simulink model "afe_rst_inv_psm_distributed_control_two_delays"  (R2025b)
settings: Solver=ode1be  StartTime=0.0  StopTime=simlength  FixedStep=tc  MaxStep=Tc
undefined symbols (not defined in the file): Adrso, Amplitude_U, Amplitude_V, Amplitude_W, Aresd, b, Bresd, CFi, CFu, Cresd, Crso, CTRPIFF_CLIP_RELEASE, dead_time_INV, emf_fb_p, emf_fb_p_ccaller_1, emf_fb_p_ccaller_2, emf_p, emf_p_ccaller_1, emf_p_ccaller_2, end_time_LVRT, fPWM_INV, g0_161Hz, g0_500Hz, g1_161Hz, g1_500Hz, i_grid_neg_eta_lim, i_grid_neg_eta_red_lim, i_grid_neg_xi_lim, i_grid_neg_xi_red_lim, i_grid_pos_eta_lim, i_grid_pos_eta_red_lim, ibez, id_lim, ieta_neg_ref_lim, ieta_pos_ref_lim, Igrid_phase_normalization_factor, iq_lim, ixi_pos_ref_lim, Jm, Jm_norm, k_frt_ref, kg, ki_afe, ki_i, ki_id, ki_iq, ki_rc_neg_grid, ki_rc_pos_grid, ki_vs, ki_w, kp_afe, kp_i, kp_id, kp_iq, kp_rc_neg_grid, kp_rc_pos_grid, kp_vs, kp_w, kw, l1 ... (+47)
libraries: fl_lib x145, nesl_utility x81, simulink x11, cstblocks x7, single_phase_transformer_lib x3, flexshaft_lib x1, pmsm_uvw_with_harmonics_lib x1
(part 8 of 15)

== system afe_rst_inv_psm_distributed_control_two_delays/mainboard_afe/voltage_sequence_avg/Moving Average Filter2/Reset Trigger ==
  Clock : Clock
  Constant1 : Constant  Value=simlength
  Constant3 : Constant  Value=0
  Constant4 : Constant
  Mod : Math  Operator=mod
  Switch : Switch  Criteria=u2 ~= 0  SaturateOnIntegerOverflow=off  InputSameDT=off
  Zero-Order Hold : ZeroOrderHold  SampleTime=ts_afe
  Out1 : Outport
  wires:
  Constant3/1 -> Switch/1
  Zero-Order Hold/1 -> Mod/1
  Constant4/1 -> Switch/3
  Mod/1 -> Switch/2
  Clock/1 -> Zero-Order Hold/1
  Switch/1 -> Out1/1  "Reset"
  Constant1/1 -> Mod/2

== system afe_rst_inv_psm_distributed_control_two_delays/mainboard_afe/voltage_sequence_avg/Moving Average Filter3/Enabled Subsystem ==
  In1 : Inport
  Enable : EnablePort
  Constant2 : Constant
  Divide : Product  Inputs=*/
  Gain1 : Gain  Gain=1/(2*pi)
  Gain9 : Gain  Gain=2
  Zero-Order Hold : ZeroOrderHold  SampleTime=ts_afe
  Out1 : Outport
  wires:
  Gain1/1 -> Gain9/1
  Zero-Order Hold/1 -> Out1/1  "period"
  Gain9/1 -> Divide/2
  In1/1 -> Gain1/1  "Omega_el"
  Divide/1 -> Zero-Order Hold/1
  Constant2/1 -> Divide/1

== system afe_rst_inv_psm_distributed_control_two_delays/mainboard_afe/voltage_sequence_avg/Moving Average Filter3/Reset Trigger ==
  Clock : Clock
  Constant1 : Constant  Value=simlength
  Constant3 : Constant  Value=0
  Constant4 : Constant
  Mod : Math  Operator=mod
  Switch : Switch  Criteria=u2 ~= 0  SaturateOnIntegerOverflow=off  InputSameDT=off
  Zero-Order Hold : ZeroOrderHold  SampleTime=ts_afe
  Out1 : Outport
  wires:
  Constant1/1 -> Mod/2
  Switch/1 -> Out1/1  "Reset"
  Clock/1 -> Zero-Order Hold/1
  Mod/1 -> Switch/2
  Constant4/1 -> Switch/3
  Zero-Order Hold/1 -> Mod/1
  Constant3/1 -> Switch/1

== system afe_rst_inv_psm_distributed_control_two_delays/mainboard_afe/voltage_sequence_avg/Moving Average Filter4/Enabled Subsystem ==
  In1 : Inport
  Enable : EnablePort
  Constant2 : Constant
  Divide : Product  Inputs=*/
  Gain1 : Gain  Gain=1/(2*pi)
  Gain9 : Gain  Gain=2
  Zero-Order Hold : ZeroOrderHold  SampleTime=ts_afe
  Out1 : Outport
  wires:
  Constant2/1 -> Divide/1
  Divide/1 -> Zero-Order Hold/1
  In1/1 -> Gain1/1  "Omega_el"
  Gain9/1 -> Divide/2
  Zero-Order Hold/1 -> Out1/1  "period"
  Gain1/1 -> Gain9/1

== system afe_rst_inv_psm_distributed_control_two_delays/mainboard_afe/voltage_sequence_avg/Moving Average Filter4/Reset Trigger ==
  Clock : Clock
  Constant1 : Constant  Value=simlength
  Constant3 : Constant  Value=0
  Constant4 : Constant
  Mod : Math  Operator=mod
  Switch : Switch  Criteria=u2 ~= 0  SaturateOnIntegerOverflow=off  InputSameDT=off
  Zero-Order Hold : ZeroOrderHold  SampleTime=ts_afe
  Out1 : Outport
  wires:
  Constant3/1 -> Switch/1
  Zero-Order Hold/1 -> Mod/1
  Constant4/1 -> Switch/3
  Mod/1 -> Switch/2
  Clock/1 -> Zero-Order Hold/1
  Switch/1 -> Out1/1  "Reset"
  Constant1/1 -> Mod/2

== system afe_rst_inv_psm_distributed_control_two_delays/AFE-Modular/afe_leg_a/driver_board_a/current_ctrl/phase_current_control ==
  In1 : Inport
  is_abc : Inport  Port=2
  Bus Creator1 : BusCreator  Inputs=2
  Bus Creator2 : BusCreator  Inputs=3
  Bus Selector1 : BusSelector  OutputSignals=usa_ctrl,usb_ctrl,usc_ctrl
  MATLAB Function : MATLAB Function  TreatAsAtomicUnit=on
  Selector : Selector  InputPortWidth=3  IndexOptions=Index vector (dialog)  Indices=1  OutputSizes=1
  Unit Delay2 : UnitDelay  SampleTime=ts_afe  HasFrameUpgradeWarning=on
  Unit Delay3 : UnitDelay  SampleTime=ts_afe  HasFrameUpgradeWarning=on
  isa_ref/isa : Scope  NumInputPorts=2
      settings: SampleTime=ts_afe  ActiveDisplayYMinimum=-1.14664  ActiveDisplayYMaximum=1.21003
  phase-current-control-dba : Subsystem
  us_alphabeta_ctrl : Outport  VectorParamsAs1DForOutWhenUnconnected=off
  tag scope: usa_ctrl_dba=global
  wires:
  Bus Creator1/1 -> us_alphabeta_ctrl/1
  Unit Delay2/1 -> Bus Creator1/1  "us_alpha_ctrl"
  Bus Selector1/1 -> MATLAB Function/1(a)  "<usa_ctrl>"
  MATLAB Function/2(beta) -> Unit Delay3/1
  Bus Selector1/2 -> MATLAB Function/2(b)  "<usb_ctrl>"
  Unit Delay3/1 -> Bus Creator1/2  "us_beta_ctrl"
  MATLAB Function/1(alpha) -> Unit Delay2/1
  Bus Selector1/3 -> MATLAB Function/3(c)  "<usc_ctrl>"
  phase-current-control-dba/1(Out1) -> [usa_ctrl_dba], Bus Creator2/1  "usa_ctrl"
  is_abc/1 -> phase-current-control-dba/2(is_abc), isa_ref/isa/2  "isa"
  In1/1 -> Selector/1
  [usb_ctrl_dbb_fb_dba] -> Bus Creator2/2  "usb_ctrl"
  [usc_ctrl_dbc_fb_dba] -> Bus Creator2/3  "usc_ctrl"
  Bus Creator2/1 -> Bus Selector1/1  "us_abc_ctrl"
  Selector/1 -> phase-current-control-dba/1(In1), isa_ref/isa/1  "isa_ref"

== system afe_rst_inv_psm_distributed_control_two_delays/AFE-Modular/afe_leg_a/driver_board_a/current_ctrl/xieta2abc ==
  pos_xi : Inport
  pos_eta : Inport  Port=2
  neg_xi : Inport  Port=3
  neg_eta : Inport  Port=4
  gamma : Inport  Port=5
  MATLAB Function2 : MATLAB Function  TreatAsAtomicUnit=on
  Mux : Mux  Inputs=3
  Negative Sequence : MATLAB Function  TreatAsAtomicUnit=on
  Positive Sequence : MATLAB Function  TreatAsAtomicUnit=on
  Sum : Sum  Inputs=|++
  Sum1 : Sum  Inputs=|++
  i_abc : Outport
  wires:
  Mux/1 -> i_abc/1  "i_abc"
  pos_eta/1 -> Positive Sequence/2(eta)
  pos_xi/1 -> Positive Sequence/1(xi)
  neg_xi/1 -> Negative Sequence/1(xi)
  Sum1/1 -> MATLAB Function2/2(beta)
  MATLAB Function2/2(b) -> Mux/2  "i_b"
  Negative Sequence/2(beta) -> Sum1/2
  Positive Sequence/1(alpha) -> Sum/1
  Negative Sequence/1(alpha) -> Sum/2
  MATLAB Function2/3(c) -> Mux/3  "i_c"
  gamma/1 -> Positive Sequence/3(gamma), Negative Sequence/3(gamma)
  Sum/1 -> MATLAB Function2/1(alpha)
  Positive Sequence/2(beta) -> Sum1/1
  MATLAB Function2/1(a) -> Mux/1  "i_a"
  neg_eta/1 -> Negative Sequence/2(eta)

== system afe_rst_inv_psm_distributed_control_two_delays/AFE-Modular/afe_leg_a/driver_board_a/dq_pll/pll_stageA ==
  gamma_grid : Inport
  Math Function : Math  Operator=magnitude^2  SignedPower=on
  Math Function1 : Math  Operator=magnitude^2  SignedPower=on
  Reciprocal Sqrt : Sqrt  Operator=rSqrt
  Saturation : Saturate  UpperLimit=inf  LowerLimit=0.02
  Sum : Sum  Inputs=|++
  sequences : Subsystem
  transformation : Subsystem
  u_grid_pos_xi : Outport  VectorParamsAs1DForOutWhenUnconnected=off
  u_grid_pos_eta : Outport  Port=2  VectorParamsAs1DForOutWhenUnconnected=off
  tag scope: ugrid_unorm_phase_a=global
  wires:
  transformation/1(ug_alpha) -> Math Function/1, sequences/1(u_grid_alpha)
  transformation/2(ug_beta) -> Math Function1/1, sequences/2(u_grid_beta)
  Math Function/1 -> Sum/1
  Math Function1/1 -> Sum/2
  Sum/1 -> Saturation/1
  Reciprocal Sqrt/1 -> [ugrid_unorm_phase_a]
  Saturation/1 -> Reciprocal Sqrt/1
  gamma_grid/1 -> sequences/3(gamma_grid)
  sequences/1(u_grid_pos_xi) -> u_grid_pos_xi/1
  sequences/2(u_grid_pos_eta) -> u_grid_pos_eta/1
  [ugb_pu_dbb_fb_dba] -> transformation/2(ug_b)
  [uga_pu_dba] -> transformation/1(ug_a)
  [ugc_pu_dbc_fb_dba] -> transformation/3(ug_c)

== system afe_rst_inv_psm_distributed_control_two_delays/AFE-Modular/afe_leg_a/driver_board_a/dq_pll/pll_stageB ==
  u_grid_pos_xi : Inport
  u_grid_pos_eta : Inport  Port=2
  -2<x<2 : Saturate  UpperLimit=2  LowerLimit=-2
  Constant4 : Constant  Value=omega_grid_nom
  Product1 : Product  RndMeth=Zero
  Product2 : Product  RndMeth=Zero
  Sum3 : Sum  SaturateOnIntegerOverflow=on
  Sum4 : Sum  SaturateOnIntegerOverflow=on
  Sum5 : Sum  Inputs=++|
  Unit Delay{1..5} (5 alike) : UnitDelay  SampleTime=ts_afe  HasFrameUpgradeWarning=on
  bounder1 : MATLAB Function  TreatAsAtomicUnit=on  SystemSampleTime=ts_afe
  kp : Gain  Gain=pll_i1*ts_afe  SaturateOnIntegerOverflow=on  OutDataTypeStr=Inherit: Same as input  ParamDataTypeStr=Inherit: Same as input
  kp1 : Gain  Gain=pll_p  SaturateOnIntegerOverflow=on  OutDataTypeStr=Inherit: Same as input  ParamDataTypeStr=Inherit: Same as input
  kp2 : Gain  Gain=ts_afe  SaturateOnIntegerOverflow=on  OutDataTypeStr=Inherit: Same as input  ParamDataTypeStr=Inherit: Same as input
  gamma_grid_pll : Outport  VectorParamsAs1DForOutWhenUnconnected=off
  wires:
  Unit Delay4/1 -> Sum5/2, Sum3/2
  Sum3/1 -> -2<x<2/1
  Sum4/1 -> bounder1/1(u)
  Unit Delay1/1 -> Sum4/2
  -2<x<2/1 -> Unit Delay4/1  "i1"
  kp2/1 -> Sum4/1
  Constant4/1 -> Product2/2
  [ugrid_unorm_phase_a] -> Unit Delay3/1
  kp/1 -> Sum3/1
  Sum5/1 -> Product2/1
  bounder1/1(y) -> Unit Delay1/1, Unit Delay2/1
  u_grid_pos_eta/1 -> Unit Delay5/1
  Product2/1 -> kp2/1
  Product1/1 -> kp/1, kp1/1  "V l"
  kp1/1 -> Sum5/1
  Unit Delay2/1 -> gamma_grid_pll/1
  Unit Delay3/1 -> Product1/2
  Unit Delay5/1 -> Product1/1

== system afe_rst_inv_psm_distributed_control_two_delays/AFE-Modular/afe_leg_a/driver_board_a/voltage-current-acquisition/is_eta_neg_ref_fieldbus ==
  is : Inport
  Unit Delay : UnitDelay  SampleTime=ts_afe  HasFrameUpgradeWarning=on
  Unit Delay1 : UnitDelay  SampleTime=ts_afe  HasFrameUpgradeWarning=on
  Zero-Order Hold : ZeroOrderHold  SampleTime=ts_afe
  is_fb : Outport
  wires:
  is/1 -> Zero-Order Hold/1
  Unit Delay/1 -> Unit Delay1/1
  Zero-Order Hold/1 -> Unit Delay/1
  Unit Delay1/1 -> is_fb/1

== system afe_rst_inv_psm_distributed_control_two_delays/AFE-Modular/afe_leg_a/driver_board_a/voltage-current-acquisition/is_eta_pos_ref_fieldbus ==
  is : Inport
  Unit Delay : UnitDelay  SampleTime=ts_afe  HasFrameUpgradeWarning=on
  Unit Delay1 : UnitDelay  SampleTime=ts_afe  HasFrameUpgradeWarning=on
  Zero-Order Hold : ZeroOrderHold  SampleTime=ts_afe
  is_fb : Outport
  wires:
  is/1 -> Zero-Order Hold/1
  Unit Delay/1 -> Unit Delay1/1
  Zero-Order Hold/1 -> Unit Delay/1
  Unit Delay1/1 -> is_fb/1

== system afe_rst_inv_psm_distributed_control_two_delays/AFE-Modular/afe_leg_a/driver_board_a/voltage-current-acquisition/is_xi_neg_ref_fieldbus ==
  is : Inport
  Unit Delay : UnitDelay  SampleTime=ts_afe  HasFrameUpgradeWarning=on
  Unit Delay1 : UnitDelay  SampleTime=ts_afe  HasFrameUpgradeWarning=on
  Zero-Order Hold : ZeroOrderHold  SampleTime=ts_afe
  is_fb : Outport
  wires:
  Unit Delay/1 -> Unit Delay1/1
  Zero-Order Hold/1 -> Unit Delay/1
  is/1 -> Zero-Order Hold/1
  Unit Delay1/1 -> is_fb/1

== system afe_rst_inv_psm_distributed_control_two_delays/AFE-Modular/afe_leg_a/driver_board_a/voltage-current-acquisition/isa_measure ==
  is : Inport
  Gain : Gain  Gain=1/Igrid_phase_normalization_factor
  Quantizer : Quantizer  QuantizationInterval=CurrentQuantization
  Unit Delay : UnitDelay  SampleTime=ts_afe  HasFrameUpgradeWarning=on
  Zero-Order Hold : ZeroOrderHold  SampleTime=ts_afe
  is_pu : Outport
  wires:
  Quantizer/1 -> Zero-Order Hold/1
  Gain/1 -> is_pu/1
  Zero-Order Hold/1 -> Unit Delay/1
  Unit Delay/1 -> Gain/1
  is/1 -> Quantizer/1

== system afe_rst_inv_psm_distributed_control_two_delays/AFE-Modular/afe_leg_a/driver_board_a/voltage-current-acquisition/isb_fieldbus ==
  is : Inport
  Unit Delay : UnitDelay  SampleTime=ts_afe  HasFrameUpgradeWarning=on
  Unit Delay1 : UnitDelay  SampleTime=ts_afe  HasFrameUpgradeWarning=on
  Zero-Order Hold : ZeroOrderHold  SampleTime=ts_afe
  is_fb : Outport
  wires:
  is/1 -> Zero-Order Hold/1
  Unit Delay/1 -> Unit Delay1/1
  Zero-Order Hold/1 -> Unit Delay/1
  Unit Delay1/1 -> is_fb/1

== system afe_rst_inv_psm_distributed_control_two_delays/AFE-Modular/afe_leg_a/driver_board_a/voltage-current-acquisition/isc_fieldbus ==
  is : Inport
  Unit Delay : UnitDelay  SampleTime=ts_afe  HasFrameUpgradeWarning=on
  Unit Delay1 : UnitDelay  SampleTime=ts_afe  HasFrameUpgradeWarning=on
  Zero-Order Hold : ZeroOrderHold  SampleTime=ts_afe
  is_fb : Outport
  wires:
  is/1 -> Zero-Order Hold/1
  Unit Delay/1 -> Unit Delay1/1
  Zero-Order Hold/1 -> Unit Delay/1
  Unit Delay1/1 -> is_fb/1

== system afe_rst_inv_psm_distributed_control_two_delays/AFE-Modular/afe_leg_a/driver_board_a/voltage-current-acquisition/ixi_ref_fieldbus ==
  is : Inport
  Unit Delay : UnitDelay  SampleTime=ts_afe  HasFrameUpgradeWarning=on
  Unit Delay1 : UnitDelay  SampleTime=ts_afe  HasFrameUpgradeWarning=on
  Zero-Order Hold : ZeroOrderHold  SampleTime=ts_afe
  is_fb : Outport
  wires:
  is/1 -> Zero-Order Hold/1
  Unit Delay/1 -> Unit Delay1/1
  Zero-Order Hold/1 -> Unit Delay/1
  Unit Delay1/1 -> is_fb/1

== system afe_rst_inv_psm_distributed_control_two_delays/AFE-Modular/afe_leg_a/driver_board_a/voltage-current-acquisition/ixi_ref_fieldbus1 ==
  is : Inport
  Unit Delay : UnitDelay  SampleTime=ts_afe  HasFrameUpgradeWarning=on
  Unit Delay1 : UnitDelay  SampleTime=ts_afe  HasFrameUpgradeWarning=on
  Zero-Order Hold : ZeroOrderHold  SampleTime=ts_afe
  is_fb : Outport
  wires:
  is/1 -> Zero-Order Hold/1
  Unit Delay/1 -> Unit Delay1/1
  Zero-Order Hold/1 -> Unit Delay/1
  Unit Delay1/1 -> is_fb/1

== system afe_rst_inv_psm_distributed_control_two_delays/AFE-Modular/afe_leg_a/driver_board_a/voltage-current-acquisition/ub_ctrl_fieldbus ==
  u_ctrl : Inport
  Unit Delay : UnitDelay  SampleTime=ts_afe  HasFrameUpgradeWarning=on
  Unit Delay1 : UnitDelay  SampleTime=ts_afe  HasFrameUpgradeWarning=on
  Zero-Order Hold : ZeroOrderHold  SampleTime=ts_afe
  u_ctrl_fb : Outport
  wires:
  u_ctrl/1 -> Zero-Order Hold/1
  Unit Delay/1 -> Unit Delay1/1
  Zero-Order Hold/1 -> Unit Delay/1
  Unit Delay1/1 -> u_ctrl_fb/1

== system afe_rst_inv_psm_distributed_control_two_delays/AFE-Modular/afe_leg_a/driver_board_a/voltage-current-acquisition/uc_ctrl_fieldbus ==
  u_ctrl : Inport
  Unit Delay : UnitDelay  SampleTime=ts_afe  HasFrameUpgradeWarning=on
  Unit Delay1 : UnitDelay  SampleTime=ts_afe  HasFrameUpgradeWarning=on
  Zero-Order Hold : ZeroOrderHold  SampleTime=ts_afe
  u_ctrl_fb : Outport
  wires:
  Zero-Order Hold/1 -> Unit Delay/1
  u_ctrl/1 -> Zero-Order Hold/1
  Unit Delay/1 -> Unit Delay1/1
  Unit Delay1/1 -> u_ctrl_fb/1

== system afe_rst_inv_psm_distributed_control_two_delays/AFE-Modular/afe_leg_a/driver_board_a/voltage-current-acquisition/uga_measure ==
  ug : Inport
  Gain : Gain  Gain=1/V_phase_normalization_factor
  Quantizer : Quantizer  QuantizationInterval=CurrentQuantization
  Unit Delay : UnitDelay  SampleTime=ts_afe  HasFrameUpgradeWarning=on
  Zero-Order Hold : ZeroOrderHold  SampleTime=ts_afe
  ug_pu : Outport
  wires:
  ug/1 -> Quantizer/1
  Unit Delay/1 -> Gain/1
  Zero-Order Hold/1 -> Unit Delay/1
  Gain/1 -> ug_pu/1
  Quantizer/1 -> Zero-Order Hold/1

== system afe_rst_inv_psm_distributed_control_two_delays/AFE-Modular/afe_leg_a/driver_board_a/voltage-current-acquisition/ugb_fieldbus ==
  ug : Inport
  Unit Delay : UnitDelay  SampleTime=ts_afe  HasFrameUpgradeWarning=on
  Unit Delay1 : UnitDelay  SampleTime=ts_afe  HasFrameUpgradeWarning=on
  Zero-Order Hold : ZeroOrderHold  SampleTime=ts_afe
  ug_fb : Outport
  wires:
  ug/1 -> Zero-Order Hold/1
  Zero-Order Hold/1 -> Unit Delay/1
  Unit Delay/1 -> Unit Delay1/1
  Unit Delay1/1 -> ug_fb/1

== system afe_rst_inv_psm_distributed_control_two_delays/AFE-Modular/afe_leg_a/driver_board_a/voltage-current-acquisition/ugc_fieldbus ==
  ug : Inport
  Unit Delay : UnitDelay  SampleTime=ts_afe  HasFrameUpgradeWarning=on
  Unit Delay1 : UnitDelay  SampleTime=ts_afe  HasFrameUpgradeWarning=on
  Zero-Order Hold : ZeroOrderHold  SampleTime=ts_afe
  ug_fb : Outport
  wires:
  ug/1 -> Zero-Order Hold/1
  Unit Delay/1 -> Unit Delay1/1
  Zero-Order Hold/1 -> Unit Delay/1
  Unit Delay1/1 -> ug_fb/1

== system afe_rst_inv_psm_distributed_control_two_delays/AFE-Modular/afe_leg_a/modulator/sv_pwm/modulator ==
  u : Inport
  v : Inport  Port=2
  w : Inport  Port=3
  Bus Creator : BusCreator  Inputs=6
  PWM generator 1 : Subsystem  mask{f=fPWM_INV, ph=0, m_up=0.98, m_low=0.02, dead_time=dead_time_INV, vg_firing=15, polarity=1}
      mask prompts: f "Frequency"; ph "Phase"; m_up "Max Input Modulation Value"; m_low "Min Input Modulation Value"; dead_time "Dead Time"; vg_firing "Gate Voltage"
  PWM generator 2 : Subsystem  mask{f=fPWM_INV, ph=0, m_up=0.98, m_low=0.02, dead_time=dead_time_INV, vg_firing=15, polarity=1}
      mask prompts: f "Frequency"; ph "Phase"; m_up "Max Input Modulation Value"; m_low "Min Input Modulation Value"; dead_time "Dead Time"; vg_firing "Gate Voltage"
  PWM generator 3 : Subsystem  mask{f=fPWM_INV, ph=0, m_up=0.98, m_low=0.02, dead_time=dead_time_INV, vg_firing=15, polarity=1}
      mask prompts: f "Frequency"; ph "Phase"; m_up "Max Input Modulation Value"; m_low "Min Input Modulation Value"; dead_time "Dead Time"; vg_firing "Gate Voltage"
  firing_gates : Outport
  wires:
  u/1 -> PWM generator 1/1(m_index)
  w/1 -> PWM generator 3/1(m_index)
  v/1 -> PWM generator 2/1(m_index)
  PWM generator 1/2(m2) -> Bus Creator/2  "pwm_u_bottom"
  Bus Creator/1 -> firing_gates/1
  PWM generator 2/1(m1) -> Bus Creator/3  "pwm_v_top"
  PWM generator 3/1(m1) -> Bus Creator/5  "pwm_w_top"
  PWM generator 2/2(m2) -> Bus Creator/4  "pwm_v_bottom"
  PWM generator 3/2(m2) -> Bus Creator/6  "pwm_w_bottom"
  PWM generator 1/1(m1) -> Bus Creator/1  "pwm_u_top"

== system afe_rst_inv_psm_distributed_control_two_delays/AFE-Modular/afe_leg_b/driver_board_b/current_ctrl/phase_current_control ==
  In1 : Inport
  is_abc : Inport  Port=2
  Bus Creator1 : BusCreator  Inputs=2
  Bus Creator2 : BusCreator  Inputs=3
  Bus Selector1 : BusSelector  OutputSignals=usa_ctrl,usb_ctrl,usc_ctrl
  MATLAB Function : MATLAB Function  TreatAsAtomicUnit=on
  Selector : Selector  InputPortWidth=3  IndexOptions=Index vector (dialog)  Indices=2  OutputSizes=1
  Unit Delay2 : UnitDelay  SampleTime=ts_afe  HasFrameUpgradeWarning=on
  Unit Delay3 : UnitDelay  SampleTime=ts_afe  HasFrameUpgradeWarning=on
  isb_ref/isb : Scope  NumInputPorts=2
      settings: SampleTime=ts_afe  ActiveDisplayYMinimum=-2.19741  ActiveDisplayYMaximum=6.15124
  phase-current-control-dbb : Subsystem
  us_alphabeta_ctrl : Outport  VectorParamsAs1DForOutWhenUnconnected=off
  tag scope: usb_ctrl_dbb=global
  wires:
  Bus Creator1/1 -> us_alphabeta_ctrl/1
  Unit Delay2/1 -> Bus Creator1/1  "us_alpha_ctrl"
  Bus Selector1/1 -> MATLAB Function/1(a)  "<usa_ctrl>"
  MATLAB Function/2(beta) -> Unit Delay3/1
  Bus Selector1/2 -> MATLAB Function/2(b)  "<usb_ctrl>"
  Unit Delay3/1 -> Bus Creator1/2  "us_beta_ctrl"
  MATLAB Function/1(alpha) -> Unit Delay2/1
  Bus Selector1/3 -> MATLAB Function/3(c)  "<usc_ctrl>"
  is_abc/1 -> phase-current-control-dbb/2(is_abc), isb_ref/isb/2  "isb"
  In1/1 -> Selector/1
  [usc_ctrl_dbc_fb_dbb] -> Bus Creator2/3  "usc_ctrl"
  phase-current-control-dbb/1(Out1) -> [usb_ctrl_dbb], Bus Creator2/2  "usb_ctrl"
  [usa_ctrl_dba_fb_dbb] -> Bus Creator2/1  "usa_ctrl"
  Bus Creator2/1 -> Bus Selector1/1  "us_abc_ctrl"
  Selector/1 -> phase-current-control-dbb/1(In1), isb_ref/isb/1  "isb_ref"

== system afe_rst_inv_psm_distributed_control_two_delays/AFE-Modular/afe_leg_b/driver_board_b/current_ctrl/xieta2abc ==
  pos_xi : Inport
  pos_eta : Inport  Port=2
  neg_xi : Inport  Port=3
  neg_eta : Inport  Port=4
  gamma : Inport  Port=5
  MATLAB Function2 : MATLAB Function  TreatAsAtomicUnit=on
  Mux : Mux  Inputs=3
  Negative Sequence : MATLAB Function  TreatAsAtomicUnit=on
  Positive Sequence : MATLAB Function  TreatAsAtomicUnit=on
  Sum : Sum  Inputs=|++
  Sum1 : Sum  Inputs=|++
  i_abc_reference : Outport
  wires:
  Mux/1 -> i_abc_reference/1  "i_abc_reference"
  pos_eta/1 -> Positive Sequence/2(eta)
  pos_xi/1 -> Positive Sequence/1(xi)
  neg_xi/1 -> Negative Sequence/1(xi)
  Sum1/1 -> MATLAB Function2/2(beta)
  MATLAB Function2/2(b) -> Mux/2  "i_b"
  Negative Sequence/2(beta) -> Sum1/2
  Positive Sequence/1(alpha) -> Sum/1
  Negative Sequence/1(alpha) -> Sum/2
  MATLAB Function2/3(c) -> Mux/3  "i_c"
  gamma/1 -> Positive Sequence/3(gamma), Negative Sequence/3(gamma)
  Sum/1 -> MATLAB Function2/1(alpha)
  Positive Sequence/2(beta) -> Sum1/1
  MATLAB Function2/1(a) -> Mux/1  "i_a"
  neg_eta/1 -> Negative Sequence/2(eta)

== system afe_rst_inv_psm_distributed_control_two_delays/AFE-Modular/afe_leg_b/driver_board_b/dq_pll/pll_stageA ==
  gamma_grid : Inport
  Math Function : Math  Operator=magnitude^2  SignedPower=on
  Math Function1 : Math  Operator=magnitude^2  SignedPower=on
  Reciprocal Sqrt : Sqrt  Operator=rSqrt
  Saturation : Saturate  UpperLimit=inf  LowerLimit=0.02
  Sum : Sum  Inputs=|++
  mormalization_and_transformation : Subsystem
  sequences : Subsystem
  u_grid_pos_xi : Outport  VectorParamsAs1DForOutWhenUnconnected=off
  u_grid_pos_eta : Outport  Port=2  VectorParamsAs1DForOutWhenUnconnected=off
  tag scope: ugrid_unorm_phase_b=global
  wires:
  mormalization_and_transformation/1(ug_alpha) -> Math Function/1, sequences/1(u_grid_alpha)
  mormalization_and_transformation/2(ug_beta) -> Math Function1/1, sequences/2(u_grid_beta)
  Math Function/1 -> Sum/1
  Math Function1/1 -> Sum/2
  Sum/1 -> Saturation/1
  Reciprocal Sqrt/1 -> [ugrid_unorm_phase_b]
  Saturation/1 -> Reciprocal Sqrt/1
  gamma_grid/1 -> sequences/3(gamma_grid)
  sequences/1(u_grid_pos_xi) -> u_grid_pos_xi/1
  sequences/2(u_grid_pos_eta) -> u_grid_pos_eta/1
  [ugb_pu_dbb] -> mormalization_and_transformation/2(ug_b)
  [uga_pu_dba_fb_dbb] -> mormalization_and_transformation/1(ug_a)
  [ugc_pu_dbc_fb_dbb] -> mormalization_and_transformation/3(ug_c)

== system afe_rst_inv_psm_distributed_control_two_delays/AFE-Modular/afe_leg_b/driver_board_b/dq_pll/pll_stageB ==
  u_grid_pos_xi : Inport
  u_grid_pos_eta : Inport  Port=2
  -2<x<2 : Saturate  UpperLimit=2  LowerLimit=-2
  Constant4 : Constant  Value=omega_grid_nom
  Product1 : Product  RndMeth=Zero
  Product2 : Product  RndMeth=Zero
  Sum3 : Sum  SaturateOnIntegerOverflow=on
  Sum4 : Sum  SaturateOnIntegerOverflow=on
  Sum5 : Sum  Inputs=++|
  Unit Delay{1..4} (4 alike) : UnitDelay  SampleTime=ts_afe  HasFrameUpgradeWarning=on
  bounder1 : MATLAB Function  TreatAsAtomicUnit=on  SystemSampleTime=ts_afe
  kp : Gain  Gain=pll_i1*ts_afe  SaturateOnIntegerOverflow=on  OutDataTypeStr=Inherit: Same as input  ParamDataTypeStr=Inherit: Same as input
  kp1 : Gain  Gain=pll_p  SaturateOnIntegerOverflow=on  OutDataTypeStr=Inherit: Same as input  ParamDataTypeStr=Inherit: Same as input
  kp2 : Gain  Gain=ts_afe  SaturateOnIntegerOverflow=on  OutDataTypeStr=Inherit: Same as input  ParamDataTypeStr=Inherit: Same as input
  gamma_grid_pll : Outport  VectorParamsAs1DForOutWhenUnconnected=off
  wires:
  Unit Delay4/1 -> Sum5/2, Sum3/2
  Sum3/1 -> -2<x<2/1
  Sum4/1 -> bounder1/1(u)
  Unit Delay1/1 -> Sum4/2
  -2<x<2/1 -> Unit Delay4/1  "i1"
  kp2/1 -> Sum4/1
  Constant4/1 -> Product2/2
  [ugrid_unorm_phase_b] -> Unit Delay2/1
  kp/1 -> Sum3/1
  Sum5/1 -> Product2/1
  u_grid_pos_eta/1 -> Unit Delay3/1
  Product2/1 -> kp2/1
  Product1/1 -> kp/1, kp1/1  "V l"
  kp1/1 -> Sum5/1
  bounder1/1(y) -> gamma_grid_pll/1, Unit Delay1/1
  Unit Delay2/1 -> Product1/2
  Unit Delay3/1 -> Product1/1

== system afe_rst_inv_psm_distributed_control_two_delays/AFE-Modular/afe_leg_b/driver_board_b/voltage-current-acquisition/is_eta_neg_ref_fieldbus ==
  is : Inport
  Unit Delay : UnitDelay  SampleTime=ts_afe  HasFrameUpgradeWarning=on
  Unit Delay1 : UnitDelay  SampleTime=ts_afe  HasFrameUpgradeWarning=on
  Zero-Order Hold : ZeroOrderHold  SampleTime=ts_afe
  is_fb : Outport
  wires:
  is/1 -> Zero-Order Hold/1
  Unit Delay/1 -> Unit Delay1/1
  Zero-Order Hold/1 -> Unit Delay/1
  Unit Delay1/1 -> is_fb/1

== system afe_rst_inv_psm_distributed_control_two_delays/AFE-Modular/afe_leg_b/driver_board_b/voltage-current-acquisition/is_eta_pos_ref_fieldbus ==
  is : Inport
  Unit Delay : UnitDelay  SampleTime=ts_afe  HasFrameUpgradeWarning=on
  Unit Delay1 : UnitDelay  SampleTime=ts_afe  HasFrameUpgradeWarning=on
  Zero-Order Hold : ZeroOrderHold  SampleTime=ts_afe
  is_fb : Outport
  wires:
  is/1 -> Zero-Order Hold/1
  Unit Delay/1 -> Unit Delay1/1
  Zero-Order Hold/1 -> Unit Delay/1
  Unit Delay1/1 -> is_fb/1

== system afe_rst_inv_psm_distributed_control_two_delays/AFE-Modular/afe_leg_b/driver_board_b/voltage-current-acquisition/is_xi_neg_ref_fieldbus ==
  is : Inport
  Unit Delay : UnitDelay  SampleTime=ts_afe  HasFrameUpgradeWarning=on
  Unit Delay1 : UnitDelay  SampleTime=ts_afe  HasFrameUpgradeWarning=on
  Zero-Order Hold : ZeroOrderHold  SampleTime=ts_afe
  is_fb : Outport
  wires:
  is/1 -> Zero-Order Hold/1
  Unit Delay/1 -> Unit Delay1/1
  Zero-Order Hold/1 -> Unit Delay/1
  Unit Delay1/1 -> is_fb/1

== system afe_rst_inv_psm_distributed_control_two_delays/AFE-Modular/afe_leg_b/driver_board_b/voltage-current-acquisition/isa_measure ==
  is : Inport
  Gain : Gain  Gain=1/Igrid_phase_normalization_factor
  Quantizer : Quantizer  QuantizationInterval=CurrentQuantization
  Unit Delay : UnitDelay  SampleTime=ts_afe  HasFrameUpgradeWarning=on
  Zero-Order Hold : ZeroOrderHold  SampleTime=ts_afe
  is_pu : Outport
  wires:
  Quantizer/1 -> Zero-Order Hold/1
  Gain/1 -> is_pu/1
  Zero-Order Hold/1 -> Unit Delay/1
  Unit Delay/1 -> Gain/1
  is/1 -> Quantizer/1

== system afe_rst_inv_psm_distributed_control_two_delays/AFE-Modular/afe_leg_b/driver_board_b/voltage-current-acquisition/isb_fieldbus ==
  is : Inport
  Unit Delay : UnitDelay  SampleTime=ts_afe  HasFrameUpgradeWarning=on
  Unit Delay1 : UnitDelay  SampleTime=ts_afe  HasFrameUpgradeWarning=on
  Zero-Order Hold : ZeroOrderHold  SampleTime=ts_afe
  is_fb : Outport
  wires:
  is/1 -> Zero-Order Hold/1
  Unit Delay/1 -> Unit Delay1/1
  Zero-Order Hold/1 -> Unit Delay/1
  Unit Delay1/1 -> is_fb/1

== system afe_rst_inv_psm_distributed_control_two_delays/AFE-Modular/afe_leg_b/driver_board_b/voltage-current-acquisition/isc_fieldbus ==
  is : Inport
  Unit Delay : UnitDelay  SampleTime=ts_afe  HasFrameUpgradeWarning=on
  Unit Delay1 : UnitDelay  SampleTime=ts_afe  HasFrameUpgradeWarning=on
  Zero-Order Hold : ZeroOrderHold  SampleTime=ts_afe
  is_fb : Outport
  wires:
  is/1 -> Zero-Order Hold/1
  Unit Delay/1 -> Unit Delay1/1
  Zero-Order Hold/1 -> Unit Delay/1
  Unit Delay1/1 -> is_fb/1

== system afe_rst_inv_psm_distributed_control_two_delays/AFE-Modular/afe_leg_b/driver_board_b/voltage-current-acquisition/ixi_ref_fieldbus ==
  is : Inport
  Unit Delay : UnitDelay  SampleTime=ts_afe  HasFrameUpgradeWarning=on
  Unit Delay1 : UnitDelay  SampleTime=ts_afe  HasFrameUpgradeWarning=on
  Zero-Order Hold : ZeroOrderHold  SampleTime=ts_afe
  is_fb : Outport
  wires:
  is/1 -> Zero-Order Hold/1
  Unit Delay/1 -> Unit Delay1/1
  Zero-Order Hold/1 -> Unit Delay/1
  Unit Delay1/1 -> is_fb/1

== system afe_rst_inv_psm_distributed_control_two_delays/AFE-Modular/afe_leg_b/driver_board_b/voltage-current-acquisition/ixi_ref_fieldbus1 ==
  is : Inport
  Unit Delay : UnitDelay  SampleTime=ts_afe  HasFrameUpgradeWarning=on
  Unit Delay1 : UnitDelay  SampleTime=ts_afe  HasFrameUpgradeWarning=on
  Zero-Order Hold : ZeroOrderHold  SampleTime=ts_afe
  is_fb : Outport
  wires:
  is/1 -> Zero-Order Hold/1
  Unit Delay/1 -> Unit Delay1/1
  Zero-Order Hold/1 -> Unit Delay/1
  Unit Delay1/1 -> is_fb/1

== system afe_rst_inv_psm_distributed_control_two_delays/AFE-Modular/afe_leg_b/driver_board_b/voltage-current-acquisition/ub_ctrl_fieldbus ==
  u_ctrl : Inport
  Unit Delay : UnitDelay  SampleTime=ts_afe  HasFrameUpgradeWarning=on
  Unit Delay1 : UnitDelay  SampleTime=ts_afe  HasFrameUpgradeWarning=on
  Zero-Order Hold : ZeroOrderHold  SampleTime=ts_afe
  u_ctrl_fb : Outport
  wires:
  u_ctrl/1 -> Zero-Order Hold/1
  Unit Delay/1 -> Unit Delay1/1
  Zero-Order Hold/1 -> Unit Delay/1
  Unit Delay1/1 -> u_ctrl_fb/1

== system afe_rst_inv_psm_distributed_control_two_delays/AFE-Modular/afe_leg_b/driver_board_b/voltage-current-acquisition/uc_ctrl_fieldbus ==
  u_ctrl : Inport
  Unit Delay : UnitDelay  SampleTime=ts_afe  HasFrameUpgradeWarning=on
  Unit Delay1 : UnitDelay  SampleTime=ts_afe  HasFrameUpgradeWarning=on
  Zero-Order Hold : ZeroOrderHold  SampleTime=ts_afe
  u_ctrl_fb : Outport
  wires:
  u_ctrl/1 -> Zero-Order Hold/1
  Unit Delay/1 -> Unit Delay1/1
  Zero-Order Hold/1 -> Unit Delay/1
  Unit Delay1/1 -> u_ctrl_fb/1

== system afe_rst_inv_psm_distributed_control_two_delays/AFE-Modular/afe_leg_b/driver_board_b/voltage-current-acquisition/uga_measure ==
  ug : Inport
  Gain : Gain  Gain=1/V_phase_normalization_factor
  Quantizer : Quantizer  QuantizationInterval=CurrentQuantization
  Unit Delay : UnitDelay  SampleTime=ts_afe  HasFrameUpgradeWarning=on
  Zero-Order Hold : ZeroOrderHold  SampleTime=ts_afe
  ug_pu : Outport
  wires:
  ug/1 -> Quantizer/1
  Unit Delay/1 -> Gain/1
  Zero-Order Hold/1 -> Unit Delay/1
  Gain/1 -> ug_pu/1
  Quantizer/1 -> Zero-Order Hold/1

== system afe_rst_inv_psm_distributed_control_two_delays/AFE-Modular/afe_leg_b/driver_board_b/voltage-current-acquisition/ugb_fieldbus ==
  ug : Inport
  Unit Delay : UnitDelay  SampleTime=ts_afe  HasFrameUpgradeWarning=on
  Unit Delay1 : UnitDelay  SampleTime=ts_afe  HasFrameUpgradeWarning=on
  Zero-Order Hold : ZeroOrderHold  SampleTime=ts_afe
  ug_fb : Outport
  wires:
  ug/1 -> Zero-Order Hold/1
  Unit Delay/1 -> Unit Delay1/1
  Zero-Order Hold/1 -> Unit Delay/1
  Unit Delay1/1 -> ug_fb/1

== system afe_rst_inv_psm_distributed_control_two_delays/AFE-Modular/afe_leg_b/driver_board_b/voltage-current-acquisition/ugc_fieldbus ==
  ug : Inport
  Unit Delay : UnitDelay  SampleTime=ts_afe  HasFrameUpgradeWarning=on
  Unit Delay1 : UnitDelay  SampleTime=ts_afe  HasFrameUpgradeWarning=on
  Zero-Order Hold : ZeroOrderHold  SampleTime=ts_afe
  ug_fb : Outport
  wires:
  ug/1 -> Zero-Order Hold/1
  Unit Delay/1 -> Unit Delay1/1
  Zero-Order Hold/1 -> Unit Delay/1
  Unit Delay1/1 -> ug_fb/1

== system afe_rst_inv_psm_distributed_control_two_delays/AFE-Modular/afe_leg_b/modulator/sv_pwm/modulator ==
  u : Inport
  v : Inport  Port=2
  w : Inport  Port=3
  Bus Creator : BusCreator  Inputs=6
  PWM generator 1 : Subsystem  mask{f=fPWM_INV, ph=0, m_up=0.98, m_low=0.02, dead_time=dead_time_INV, vg_firing=15, polarity=1}
      mask prompts: f "Frequency"; ph "Phase"; m_up "Max Input Modulation Value"; m_low "Min Input Modulation Value"; dead_time "Dead Time"; vg_firing "Gate Voltage"
  PWM generator 2 : Subsystem  mask{f=fPWM_INV, ph=0, m_up=0.98, m_low=0.02, dead_time=dead_time_INV, vg_firing=15, polarity=1}
      mask prompts: f "Frequency"; ph "Phase"; m_up "Max Input Modulation Value"; m_low "Min Input Modulation Value"; dead_time "Dead Time"; vg_firing "Gate Voltage"
  PWM generator 3 : Subsystem  mask{f=fPWM_INV, ph=0, m_up=0.98, m_low=0.02, dead_time=dead_time_INV, vg_firing=15, polarity=1}
      mask prompts: f "Frequency"; ph "Phase"; m_up "Max Input Modulation Value"; m_low "Min Input Modulation Value"; dead_time "Dead Time"; vg_firing "Gate Voltage"
  firing_gates : Outport
  wires:
  PWM generator 1/1(m1) -> Bus Creator/1  "pwm_u_top"
  PWM generator 3/2(m2) -> Bus Creator/6  "pwm_w_bottom"
  PWM generator 2/2(m2) -> Bus Creator/4  "pwm_v_bottom"
  PWM generator 3/1(m1) -> Bus Creator/5  "pwm_w_top"
  PWM generator 2/1(m1) -> Bus Creator/3  "pwm_v_top"
  Bus Creator/1 -> firing_gates/1
  PWM generator 1/2(m2) -> Bus Creator/2  "pwm_u_bottom"
  v/1 -> PWM generator 2/1(m_index)
  w/1 -> PWM generator 3/1(m_index)
  u/1 -> PWM generator 1/1(m_index)

== system afe_rst_inv_psm_distributed_control_two_delays/AFE-Modular/afe_leg_c/driver_board_c/current_ctrl/phase_current_control ==
  In1 : Inport
  is_abc : Inport  Port=2
  Bus Creator1 : BusCreator  Inputs=2
  Bus Creator2 : BusCreator  Inputs=3
  Bus Selector1 : BusSelector  OutputSignals=usa_ctrl,usb_ctrl,usc_ctrl
  MATLAB Function : MATLAB Function  TreatAsAtomicUnit=on
  Selector : Selector  InputPortWidth=3  IndexOptions=Index vector (dialog)  Indices=3  OutputSizes=1
  Unit Delay2 : UnitDelay  SampleTime=ts_afe  HasFrameUpgradeWarning=on
  Unit Delay3 : UnitDelay  SampleTime=ts_afe  HasFrameUpgradeWarning=on
  isc_ref/isc : Scope  NumInputPorts=2
      settings: SampleTime=ts_afe  ActiveDisplayYMinimum=-6.6016  ActiveDisplayYMaximum=2.92896
  phase-current-control-dbc : Subsystem
  us_alphabeta_ctrl : Outport  VectorParamsAs1DForOutWhenUnconnected=off
  tag scope: usc_ctrl_dbc=global
  wires:
  Bus Creator1/1 -> us_alphabeta_ctrl/1
  Unit Delay2/1 -> Bus Creator1/1  "us_alpha_ctrl"
  Bus Selector1/1 -> MATLAB Function/1(a)  "<usa_ctrl>"
  MATLAB Function/2(beta) -> Unit Delay3/1
  Bus Selector1/2 -> MATLAB Function/2(b)  "<usb_ctrl>"
  Unit Delay3/1 -> Bus Creator1/2  "us_beta_ctrl"
  MATLAB Function/1(alpha) -> Unit Delay2/1
  Bus Selector1/3 -> MATLAB Function/3(c)  "<usc_ctrl>"
  is_abc/1 -> isc_ref/isc/2, phase-current-control-dbc/2(is_abc)  "isc"
  In1/1 -> Selector/1
  phase-current-control-dbc/1(Out1) -> Bus Creator2/3, [usc_ctrl_dbc]  "usc_ctrl"
  [usb_ctrl_dbb_fb_dbc] -> Bus Creator2/2  "usb_ctrl"
  [usa_ctrl_dba_fb_dbc] -> Bus Creator2/1  "usa_ctrl"
  Bus Creator2/1 -> Bus Selector1/1  "us_abc_ctrl"
  Selector/1 -> isc_ref/isc/1, phase-current-control-dbc/1(In1)  "isc_ref"

== system afe_rst_inv_psm_distributed_control_two_delays/AFE-Modular/afe_leg_c/driver_board_c/current_ctrl/xieta2abc ==
  pos_xi : Inport
  pos_eta : Inport  Port=2
  neg_xi : Inport  Port=3
  neg_eta : Inport  Port=4
  gamma : Inport  Port=5
  MATLAB Function2 : MATLAB Function  TreatAsAtomicUnit=on
  Mux : Mux  Inputs=3
  Negative Sequence : MATLAB Function  TreatAsAtomicUnit=on
  Positive Sequence : MATLAB Function  TreatAsAtomicUnit=on
  Sum : Sum  Inputs=|++
  Sum1 : Sum  Inputs=|++
  i_abc_reference : Outport
  wires:
  Mux/1 -> i_abc_reference/1  "i_abc_reference"
  pos_eta/1 -> Positive Sequence/2(eta)
  pos_xi/1 -> Positive Sequence/1(xi)
  neg_xi/1 -> Negative Sequence/1(xi)
  Sum1/1 -> MATLAB Function2/2(beta)
  MATLAB Function2/2(b) -> Mux/2  "i_b"
  Negative Sequence/2(beta) -> Sum1/2
  Positive Sequence/1(alpha) -> Sum/1
  Negative Sequence/1(alpha) -> Sum/2
  MATLAB Function2/3(c) -> Mux/3  "i_c"
  gamma/1 -> Positive Sequence/3(gamma), Negative Sequence/3(gamma)
  Sum/1 -> MATLAB Function2/1(alpha)
  Positive Sequence/2(beta) -> Sum1/1
  MATLAB Function2/1(a) -> Mux/1  "i_a"
  neg_eta/1 -> Negative Sequence/2(eta)

== system afe_rst_inv_psm_distributed_control_two_delays/AFE-Modular/afe_leg_c/driver_board_c/dq_pll/pll_stageA ==
  gamma_grid : Inport
  Math Function : Math  Operator=magnitude^2  SignedPower=on
  Math Function1 : Math  Operator=magnitude^2  SignedPower=on
  Reciprocal Sqrt : Sqrt  Operator=rSqrt
  Saturation : Saturate  UpperLimit=inf  LowerLimit=0.02
  Sum : Sum  Inputs=|++
  mormalization_and_transformation : Subsystem
  sequences : Subsystem
  u_grid_pos_xi : Outport  VectorParamsAs1DForOutWhenUnconnected=off
  u_grid_pos_eta : Outport  Port=2  VectorParamsAs1DForOutWhenUnconnected=off
  tag scope: ugrid_unorm_phase_c=global
  wires:
  mormalization_and_transformation/1(ug_alpha) -> Math Function/1, sequences/1(u_grid_alpha)
  mormalization_and_transformation/2(ug_beta) -> Math Function1/1, sequences/2(u_grid_beta)
  Math Function/1 -> Sum/1
  Math Function1/1 -> Sum/2
  Sum/1 -> Saturation/1
  Reciprocal Sqrt/1 -> [ugrid_unorm_phase_c]
  Saturation/1 -> Reciprocal Sqrt/1
  gamma_grid/1 -> sequences/3(gamma_grid)
  sequences/1(u_grid_pos_xi) -> u_grid_pos_xi/1
  sequences/2(u_grid_pos_eta) -> u_grid_pos_eta/1
  [ugb_pu_dbb_fb_dbc] -> mormalization_and_transformation/2(ug_b)
  [uga_pu_dba_fb_dbc] -> mormalization_and_transformation/1(ug_a)
  [ugc_pu_dbc] -> mormalization_and_transformation/3(ug_c)

== system afe_rst_inv_psm_distributed_control_two_delays/AFE-Modular/afe_leg_c/driver_board_c/dq_pll/pll_stageB ==
  u_grid_pos_xi : Inport
  u_grid_pos_eta : Inport  Port=2
  -2<x<2 : Saturate  UpperLimit=2  LowerLimit=-2
  Constant4 : Constant  Value=omega_grid_nom
  Product1 : Product  RndMeth=Zero
  Product2 : Product  RndMeth=Zero
  Sum3 : Sum  SaturateOnIntegerOverflow=on
  Sum4 : Sum  SaturateOnIntegerOverflow=on
  Sum5 : Sum  Inputs=++|
  Unit Delay{1..4} (4 alike) : UnitDelay  SampleTime=ts_afe  HasFrameUpgradeWarning=on
  bounder1 : MATLAB Function  TreatAsAtomicUnit=on  SystemSampleTime=ts_afe
  kp : Gain  Gain=pll_i1*ts_afe  SaturateOnIntegerOverflow=on  OutDataTypeStr=Inherit: Same as input  ParamDataTypeStr=Inherit: Same as input
  kp1 : Gain  Gain=pll_p  SaturateOnIntegerOverflow=on  OutDataTypeStr=Inherit: Same as input  ParamDataTypeStr=Inherit: Same as input
  kp2 : Gain  Gain=ts_afe  SaturateOnIntegerOverflow=on  OutDataTypeStr=Inherit: Same as input  ParamDataTypeStr=Inherit: Same as input
  gamma_grid_pll : Outport  VectorParamsAs1DForOutWhenUnconnected=off
  wires:
  Unit Delay4/1 -> Sum3/2, Sum5/2
  Sum3/1 -> -2<x<2/1
  Sum4/1 -> bounder1/1(u)
  Unit Delay1/1 -> Sum4/2
  -2<x<2/1 -> Unit Delay4/1  "i1"
  kp2/1 -> Sum4/1
  Constant4/1 -> Product2/2
  [ugrid_unorm_phase_c] -> Unit Delay2/1
  kp/1 -> Sum3/1
  Sum5/1 -> Product2/1
  u_grid_pos_eta/1 -> Unit Delay3/1
  Product2/1 -> kp2/1
  Product1/1 -> kp/1, kp1/1  "V l"
  kp1/1 -> Sum5/1
  bounder1/1(y) -> gamma_grid_pll/1, Unit Delay1/1
  Unit Delay2/1 -> Product1/2
  Unit Delay3/1 -> Product1/1

== system afe_rst_inv_psm_distributed_control_two_delays/AFE-Modular/afe_leg_c/driver_board_c/voltage-current-acquisition/is_eta_neg_ref_fieldbus ==
  is : Inport
  Unit Delay : UnitDelay  SampleTime=ts_afe  HasFrameUpgradeWarning=on
  Unit Delay1 : UnitDelay  SampleTime=ts_afe  HasFrameUpgradeWarning=on
  Zero-Order Hold : ZeroOrderHold  SampleTime=ts_afe
  is_fb : Outport
  wires:
  is/1 -> Zero-Order Hold/1
  Unit Delay/1 -> Unit Delay1/1
  Zero-Order Hold/1 -> Unit Delay/1
  Unit Delay1/1 -> is_fb/1

== system afe_rst_inv_psm_distributed_control_two_delays/AFE-Modular/afe_leg_c/driver_board_c/voltage-current-acquisition/is_eta_pos_ref_fieldbus ==
  is : Inport
  Unit Delay : UnitDelay  SampleTime=ts_afe  HasFrameUpgradeWarning=on
  Unit Delay1 : UnitDelay  SampleTime=ts_afe  HasFrameUpgradeWarning=on
  Zero-Order Hold : ZeroOrderHold  SampleTime=ts_afe
  is_fb : Outport
  wires:
  is/1 -> Zero-Order Hold/1
  Unit Delay/1 -> Unit Delay1/1
  Zero-Order Hold/1 -> Unit Delay/1
  Unit Delay1/1 -> is_fb/1

== system afe_rst_inv_psm_distributed_control_two_delays/AFE-Modular/afe_leg_c/driver_board_c/voltage-current-acquisition/is_xi_neg_ref_fieldbus ==
  is : Inport
  Unit Delay : UnitDelay  SampleTime=ts_afe  HasFrameUpgradeWarning=on
  Unit Delay1 : UnitDelay  SampleTime=ts_afe  HasFrameUpgradeWarning=on
  Zero-Order Hold : ZeroOrderHold  SampleTime=ts_afe
  is_fb : Outport
  wires:
  is/1 -> Zero-Order Hold/1
  Unit Delay/1 -> Unit Delay1/1
  Zero-Order Hold/1 -> Unit Delay/1
  Unit Delay1/1 -> is_fb/1

== system afe_rst_inv_psm_distributed_control_two_delays/AFE-Modular/afe_leg_c/driver_board_c/voltage-current-acquisition/isb_fieldbus ==
  is : Inport
  Unit Delay : UnitDelay  SampleTime=ts_afe  HasFrameUpgradeWarning=on
  Unit Delay1 : UnitDelay  SampleTime=ts_afe  HasFrameUpgradeWarning=on
  Zero-Order Hold : ZeroOrderHold  SampleTime=ts_afe
  is_fb : Outport
  wires:
  is/1 -> Zero-Order Hold/1
  Unit Delay/1 -> Unit Delay1/1
  Zero-Order Hold/1 -> Unit Delay/1
  Unit Delay1/1 -> is_fb/1

== system afe_rst_inv_psm_distributed_control_two_delays/AFE-Modular/afe_leg_c/driver_board_c/voltage-current-acquisition/isc_fieldbus ==
  is : Inport
  Unit Delay : UnitDelay  SampleTime=ts_afe  HasFrameUpgradeWarning=on
  Unit Delay1 : UnitDelay  SampleTime=ts_afe  HasFrameUpgradeWarning=on
  Zero-Order Hold : ZeroOrderHold  SampleTime=ts_afe
  is_fb : Outport
  wires:
  is/1 -> Zero-Order Hold/1
  Unit Delay/1 -> Unit Delay1/1
  Zero-Order Hold/1 -> Unit Delay/1
  Unit Delay1/1 -> is_fb/1

== system afe_rst_inv_psm_distributed_control_two_delays/AFE-Modular/afe_leg_c/driver_board_c/voltage-current-acquisition/isc_measure_and_normalization ==
  is : Inport
  Gain : Gain  Gain=1/Igrid_phase_normalization_factor
  Quantizer : Quantizer  QuantizationInterval=CurrentQuantization
  Unit Delay : UnitDelay  SampleTime=ts_afe  HasFrameUpgradeWarning=on
  Zero-Order Hold : ZeroOrderHold  SampleTime=ts_afe
  is_pu : Outport
  wires:
  Quantizer/1 -> Zero-Order Hold/1
  Gain/1 -> is_pu/1
  Zero-Order Hold/1 -> Unit Delay/1
  Unit Delay/1 -> Gain/1
  is/1 -> Quantizer/1

== system afe_rst_inv_psm_distributed_control_two_delays/AFE-Modular/afe_leg_c/driver_board_c/voltage-current-acquisition/ixi_ref_fieldbus ==
  is : Inport
  Unit Delay : UnitDelay  SampleTime=ts_afe  HasFrameUpgradeWarning=on
  Unit Delay1 : UnitDelay  SampleTime=ts_afe  HasFrameUpgradeWarning=on
  Zero-Order Hold : ZeroOrderHold  SampleTime=ts_afe
  is_fb : Outport
  wires:
  is/1 -> Zero-Order Hold/1
  Unit Delay/1 -> Unit Delay1/1
  Zero-Order Hold/1 -> Unit Delay/1
  Unit Delay1/1 -> is_fb/1

== system afe_rst_inv_psm_distributed_control_two_delays/AFE-Modular/afe_leg_c/driver_board_c/voltage-current-acquisition/ixi_ref_fieldbus1 ==
  is : Inport
  Unit Delay : UnitDelay  SampleTime=ts_afe  HasFrameUpgradeWarning=on
  Unit Delay1 : UnitDelay  SampleTime=ts_afe  HasFrameUpgradeWarning=on
  Zero-Order Hold : ZeroOrderHold  SampleTime=ts_afe
  is_fb : Outport
  wires:
  is/1 -> Zero-Order Hold/1
  Unit Delay/1 -> Unit Delay1/1
  Zero-Order Hold/1 -> Unit Delay/1
  Unit Delay1/1 -> is_fb/1

== system afe_rst_inv_psm_distributed_control_two_delays/AFE-Modular/afe_leg_c/driver_board_c/voltage-current-acquisition/ub_ctrl_fieldbus ==
  u_ctrl : Inport
  Unit Delay : UnitDelay  SampleTime=ts_afe  HasFrameUpgradeWarning=on
  Unit Delay1 : UnitDelay  SampleTime=ts_afe  HasFrameUpgradeWarning=on
  Zero-Order Hold : ZeroOrderHold  SampleTime=ts_afe
  u_ctrl_fb : Outport
  wires:
  u_ctrl/1 -> Zero-Order Hold/1
  Unit Delay/1 -> Unit Delay1/1
  Zero-Order Hold/1 -> Unit Delay/1
  Unit Delay1/1 -> u_ctrl_fb/1

== system afe_rst_inv_psm_distributed_control_two_delays/AFE-Modular/afe_leg_c/driver_board_c/voltage-current-acquisition/uc_ctrl_fieldbus ==
  u_ctrl : Inport
  Unit Delay : UnitDelay  SampleTime=ts_afe  HasFrameUpgradeWarning=on
  Unit Delay1 : UnitDelay  SampleTime=ts_afe  HasFrameUpgradeWarning=on
  Zero-Order Hold : ZeroOrderHold  SampleTime=ts_afe
  u_ctrl_fb : Outport
  wires:
  u_ctrl/1 -> Zero-Order Hold/1
  Unit Delay/1 -> Unit Delay1/1
  Zero-Order Hold/1 -> Unit Delay/1
  Unit Delay1/1 -> u_ctrl_fb/1

== system afe_rst_inv_psm_distributed_control_two_delays/AFE-Modular/afe_leg_c/driver_board_c/voltage-current-acquisition/uga_fieldbus ==
  ug : Inport
  Unit Delay : UnitDelay  SampleTime=ts_afe  HasFrameUpgradeWarning=on
  Unit Delay1 : UnitDelay  SampleTime=ts_afe  HasFrameUpgradeWarning=on
  Zero-Order Hold : ZeroOrderHold  SampleTime=ts_afe
  ug_fb : Outport
  wires:
  ug/1 -> Zero-Order Hold/1
  Zero-Order Hold/1 -> Unit Delay/1
  Unit Delay/1 -> Unit Delay1/1
  Unit Delay1/1 -> ug_fb/1

== system afe_rst_inv_psm_distributed_control_two_delays/AFE-Modular/afe_leg_c/driver_board_c/voltage-current-acquisition/ugb_fieldbus ==
  ug : Inport
  Unit Delay : UnitDelay  SampleTime=ts_afe  HasFrameUpgradeWarning=on
  Unit Delay1 : UnitDelay  SampleTime=ts_afe  HasFrameUpgradeWarning=on
  Zero-Order Hold : ZeroOrderHold  SampleTime=ts_afe
  ug_fb : Outport
  wires:
  ug/1 -> Zero-Order Hold/1
  Unit Delay/1 -> Unit Delay1/1
  Zero-Order Hold/1 -> Unit Delay/1
  Unit Delay1/1 -> ug_fb/1

== system afe_rst_inv_psm_distributed_control_two_delays/AFE-Modular/afe_leg_c/driver_board_c/voltage-current-acquisition/ugc_measure_and_normalization ==
  ug : Inport
  Gain : Gain  Gain=1/V_phase_normalization_factor
  Quantizer : Quantizer  QuantizationInterval=CurrentQuantization
  Unit Delay : UnitDelay  SampleTime=ts_afe  HasFrameUpgradeWarning=on
  Zero-Order Hold : ZeroOrderHold  SampleTime=ts_afe
  ug_pu : Outport
  wires:
  ug/1 -> Quantizer/1
  Unit Delay/1 -> Gain/1
  Zero-Order Hold/1 -> Unit Delay/1
  Gain/1 -> ug_pu/1
  Quantizer/1 -> Zero-Order Hold/1

== system afe_rst_inv_psm_distributed_control_two_delays/AFE-Modular/afe_leg_c/modulator/sv_pwm/modulator ==
  u : Inport
  v : Inport  Port=2
  w : Inport  Port=3
  Bus Creator : BusCreator  Inputs=6
  PWM generator 1 : Subsystem  mask{f=fPWM_INV, ph=0, m_up=0.98, m_low=0.02, dead_time=dead_time_INV, vg_firing=15, polarity=1}
      mask prompts: f "Frequency"; ph "Phase"; m_up "Max Input Modulation Value"; m_low "Min Input Modulation Value"; dead_time "Dead Time"; vg_firing "Gate Voltage"
  PWM generator 2 : Subsystem  mask{f=fPWM_INV, ph=0, m_up=0.98, m_low=0.02, dead_time=dead_time_INV, vg_firing=15, polarity=1}
      mask prompts: f "Frequency"; ph "Phase"; m_up "Max Input Modulation Value"; m_low "Min Input Modulation Value"; dead_time "Dead Time"; vg_firing "Gate Voltage"
  PWM generator 3 : Subsystem  mask{f=fPWM_INV, ph=0, m_up=0.98, m_low=0.02, dead_time=dead_time_INV, vg_firing=15, polarity=1}
      mask prompts: f "Frequency"; ph "Phase"; m_up "Max Input Modulation Value"; m_low "Min Input Modulation Value"; dead_time "Dead Time"; vg_firing "Gate Voltage"
  firing_gates : Outport
  wires:
  u/1 -> PWM generator 1/1(m_index)
  w/1 -> PWM generator 3/1(m_index)
  v/1 -> PWM generator 2/1(m_index)
  PWM generator 1/2(m2) -> Bus Creator/2  "pwm_u_bottom"
  Bus Creator/1 -> firing_gates/1
  PWM generator 2/1(m1) -> Bus Creator/3  "pwm_v_top"
  PWM generator 3/1(m1) -> Bus Creator/5  "pwm_w_top"
  PWM generator 2/2(m2) -> Bus Creator/4  "pwm_v_bottom"
  PWM generator 3/2(m2) -> Bus Creator/6  "pwm_w_bottom"
  PWM generator 1/1(m1) -> Bus Creator/1  "pwm_u_top"

== system afe_rst_inv_psm_distributed_control_two_delays/INV-Modular/inv_leg_u/driver_board_u/motor_vector_control/bemf_observer ==
  ialpha_pu : Inport
  ibeta_pu : Inport  Port=2
  ualpha_pu : Inport  Port=3
  ubeta_pu : Inport  Port=4
  Unit Delay : UnitDelay  SampleTime=ts_inv  HasFrameUpgradeWarning=on
  Unit Delay1 : UnitDelay  SampleTime=ts_inv  HasFrameUpgradeWarning=on
  bemf_observer_ccaller : Subsystem  Commented=on
  bemf_observer_simulink : Subsystem
  bemf_observer_with_load_estimator_ccaller : Subsystem  Commented=on
  tag scope: motor_omega_hat_pu_dbu=global, motor_theta_hat_dbu=global
  wires:
  ialpha_pu/1 -> bemf_observer_simulink/1(ialpha_pu)
  ibeta_pu/1 -> bemf_observer_simulink/2(ibeta_pu)
  ualpha_pu/1 -> bemf_observer_simulink/3(ualpha_pu)
  ubeta_pu/1 -> bemf_observer_simulink/4(ubeta_pu)
  bemf_observer_simulink/2(theta_hat) -> Unit Delay1/1  "theta_hat"
  bemf_observer_simulink/1(omega_pu_hat) -> Unit Delay/1  "omega_hat_pu"
  Unit Delay/1 -> [motor_omega_hat_pu_dbu]
  Unit Delay1/1 -> [motor_theta_hat_dbu]

== system afe_rst_inv_psm_distributed_control_two_delays/INV-Modular/inv_leg_u/driver_board_u/motor_vector_control/current_ctrl ==
  iq_ref : Inport
  MTPA : Subsystem
      mask Display: disp('MTPA')
  Sqrt : Sqrt
  Square : Math  Operator=square
  Square1 : Math  Operator=square
  Sum : Sum  Inputs=|++
  To Workspace7 : ToWorkspace  VariableName=u_mot_pu_sim  SampleTime=ts_inv
      settings: MaxDataPoints=Ns_inv
  dq_pi_with_vector_antiwindup : Subsystem
  id_ref : Subsystem
      settings: PortSchema="{\"entries\":[{\"content\":{\"sides\":[{\"content\":{},\"type\":\"ConnectorPlacement.EquallySpacedRectSide\",\"uuid\":\"42af5d69-f0eb-42c6-9e03-28c1d0757323\"},{\"content\":{\"connectorIds\":[\"Out1\"],\"side\":\"RIGHT\"},\"type\":\"ConnectorPlacement.EquallySpacedRectSide\",\"uuid\":\"dd68a9f9-d15f-4e57-9d9e-130889a7b90c\"},{\"content\":{\"connectorIds\":[\"In1\"],\"side\":\"TOP\"},\"type\":\"ConnectorPlacement.EquallySpacedRectSide\",\"uuid\":\"68c797a2-8439-4b8d-8368-b7485adf0676\"}]},\"type\":\"ConnectorPlacement.EquallySpacedConnector\",\"uuid\":\"693c5f1c-0580-4626-8f13-b27865dfb3ac\"}],\"packageUris\":[\"http://schema.mathworks.com/mf0/Connector/R2020b\"],\"version\":\"1.0\"}"
  idref/id : Scope  NumInputPorts=2
      settings: SampleTime=tc  ActiveDisplayYMinimum=-0.16984  ActiveDisplayYMaximum=0.0865
  iqref/iq : Scope  NumInputPorts=2
      settings: SampleTime=tc  ActiveDisplayYMinimum=-0.66775  ActiveDisplayYMaximum=0.07588  DataLoggingVariableName=ScopeData2
  ud : Outport
  uq : Outport  Port=2
  wires:
  [motor_iq_pu_dbu] -> iqref/iq/2, dq_pi_with_vector_antiwindup/4(iq)  "iq"
  [motor_id_pu_dbu] -> idref/id/2, dq_pi_with_vector_antiwindup/2(id)  "id"
  MTPA/1(Id_ref_mtpa) -> id_ref/1(id_mtpa)  "id_ref"
  dq_pi_with_vector_antiwindup/1(ctrl_d_u) -> Square1/1, ud/1
  dq_pi_with_vector_antiwindup/2(ctrl_q_u) -> Square/1, uq/1
  Square/1 -> Sum/1
  Sum/1 -> Sqrt/1
  Square1/1 -> Sum/2
  Sqrt/1 -> To Workspace7/1
  id_ref/1(id_ref) -> dq_pi_with_vector_antiwindup/1(id_ref), idref/id/1
  iq_ref/1 -> iqref/iq/1, dq_pi_with_vector_antiwindup/3(iq_ref)  "iq_ref"
  [motor_iq_pu_dbu] -> MTPA/1(iq)  "iq"
